simulink subsystem "Subsystem_Driver_DecisionMaker_BAv01"  (R2022b)
settings: Solver=VariableStepAuto  StartTime=0.0  StopTime=10.0  RelTol=1e-3
undefined symbols (not defined in the file): driver, weatherSim
settings Model: Creator=giaco  LastModifiedBy=giaco

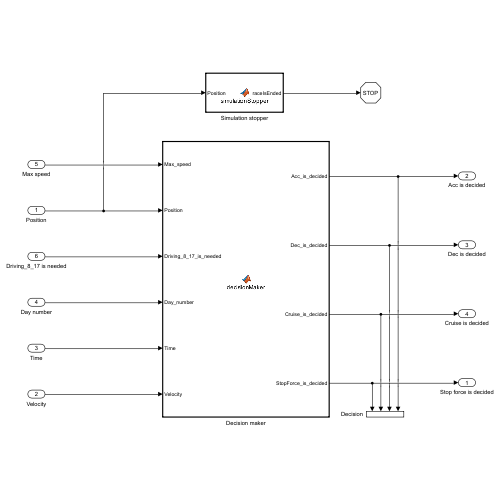
[thumbnail: Simulink's stored preview of the top-level diagram]
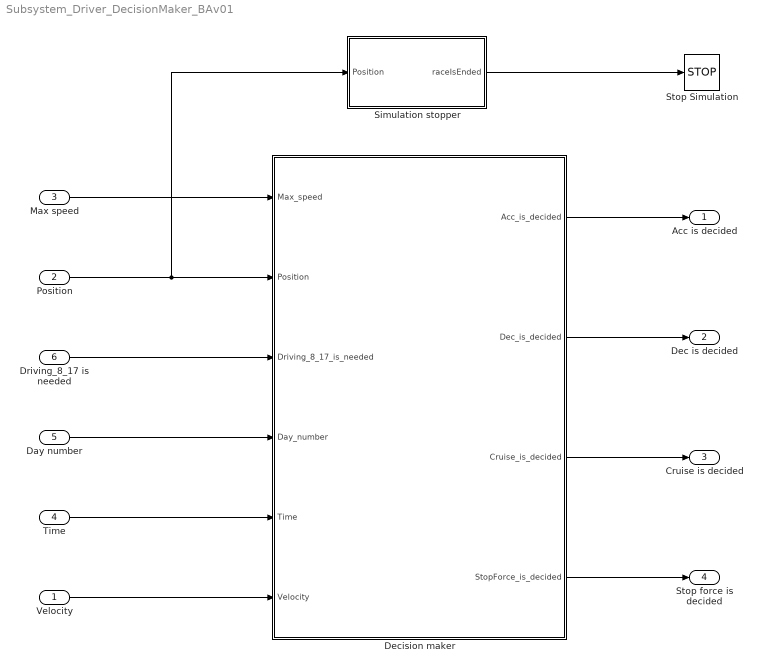
== system Subsystem_Driver_DecisionMaker_BAv01 ==
  Velocity : Inport
  Position : Inport  Port=2
  Max speed : Inport  Port=3
  Time : Inport  Port=4
  Day number : Inport  Port=5
  Driving_8_17 is needed : Inport  Port=6
  Decision maker : MATLAB Function  TreatAsAtomicUnit=on
  Simulation stopper : MATLAB Function  TreatAsAtomicUnit=on
  Stop Simulation : Stop
  Acc is decided : Outport
  Dec is decided : Outport  Port=2
  Cruise is decided : Outport  Port=3
  Stop force is decided : Outport  Port=4  OutDataTypeStr=boolean
  wires:
  Simulation stopper/1(raceIsEnded) -> Stop Simulation/1
  Velocity/1 -> Decision maker/6(Velocity)
  Driving_8_17 is needed/1 -> Decision maker/3(Driving_8_17_is_needed)
  Decision maker/3(Cruise_is_decided) -> Cruise is decided/1
  Position/1 -> Simulation stopper/1(Position), Decision maker/2(Position)
  Decision maker/2(Dec_is_decided) -> Dec is decided/1
  Time/1 -> Decision maker/5(Time)
  Decision maker/4(StopForce_is_decided) -> Stop force is decided/1
  Day number/1 -> Decision maker/4(Day_number)
  Max speed/1 -> Decision maker/1(Max_speed)
  Decision maker/1(Acc_is_decided) -> Acc is decided/1

== matlab function Subsystem_Driver_DecisionMaker_BAv01/Decision maker ==
  settings: updateMethod=DISCRETE
  data: Max_speed input; Position input; Driving_8_17_is_needed input; Day_number input; Time input; Velocity input; spaceStopIsOver data_store_memory; timeStopIsNeeded data_store_memory; spaceStopIsNeeded data_store_memory; driver parameter; spaceStopNumber data_store_memory; spaceStopIsStarted data_store_memory; Acc_is_decided output; Dec_is_decided output; Cruise_is_decided output; StopForce_is_decided output; spaceStopInitialTime data_store_memory; accInitialTime data_store_memory; accInitialVelocity data_store_memory; decInitialTime data_store_memory; decInitialVelocity data_store_memory; racingDayIsStarted data_store_memory; dayNumber data_store_memory; weatherSim parameter
function [Acc_is_decided, Dec_is_decided, Cruise_is_decided, StopForce_is_decided] = decisionMaker(Max_speed, Position, Driving_8_17_is_needed, Day_number, Time, Velocity, driver, weatherSim)

global racingDayIsStarted
global timeStopIsNeeded
global dayNumber

global spaceStopIsNeeded
global spaceStopIsStarted
global spaceStopIsOver
global spaceStopInitialTime
global spaceStopNumber

global accInitialTime
global accInitialVelocity
global decInitialTime
global decInitialVelocity

Acc_is_decided = false;
Dec_is_decided = false;
Cruise_is_decided = false;
StopForce_is_decided = false;

controlVelocity = min(driver.velRef, Max_speed);

%% Check for stops
% Time stops
stopTime = Time - Velocity ./ driver.decRef;

if ~timeStopIsNeeded && stopTime >= (weatherSim.irradiance.stopTimeSec(Day_number) - 60) %to be sure to stop on time
    timeStopIsNeeded = true;
    decInitialTime = Time; %initialization of time and velocity for ramp controller
    decInitialVelocity = Velocity;
end % if

% Space stops
stopDistance = Position - Velocity.^2 / (2 * driver.decRef);

if ~spaceStopIsNeeded && stopDistance >= driver.stopLocDist(spaceStopNumber)
    spaceStopIsNeeded = true;
    decInitialTime = Time; %initialization of time and velocity for ramp controller
    decInitialVelocity = Velocity;
    
    if spaceStopNumber < length(driver.stopLocDist) %omit last stop: stop simulation
        spaceStopNumber = spaceStopNumber + 1;
    end % if
end % if

%% Check for new racing day
if Driving_8_17_is_needed && Day_number == dayNumber
    racingDayIsStarted = true;
    timeStopIsNeeded = false;
    dayNumber = dayNumber + 1;
end % if

%% Select control options
%% Deceleration
if timeStopIsNeeded
    if Velocity > driver.velRefStop
        Dec_is_decided = true;
    else %if Velocity <= driver.velRefStop
        StopForce_is_decided = true;
        Dec_is_decided = false;
    end % if

elseif spaceStopIsNeeded
    if spaceStopIsStarted
        spaceStopDuration = Time - spaceStopInitialTime;
        if spaceStopDuration >= 30*60
            spaceStopIsNeeded = false;
            spaceStopIsStarted = false;
            spaceStopIsOver = true;
            Acc_is_decided = true;
            accInitialTime = Time;
            accInitialVelocity = Velocity;
        else
            StopForce_is_decided = true;
        end % if
    else
        if Velocity > driver.velRefStop
            Dec_is_decided = true;
        else %if Velocity < driver.velRefStop
            spaceStopIsStarted = true;
            spaceStopInitialTime = Time;
            StopForce_is_decided = true;
        end % if
    end % if

%% Acceleration
elseif racingDayIsStarted
    if Velocity < 0.9 * controlVelocity
        Acc_is_decided = true;
    else %if Velocity >= 0.9 * controlVelocity
        Cruise_is_decided = true;
        racingDayIsStarted = false;
    end % if

elseif spaceStopIsOver
    if Velocity < 0.9 * controlVelocity
        Acc_is_decided = true;
    else %if Velocity >= 0.9 * controlVelocity
        Cruise_is_decided = true;
        spaceStopIsOver = false;
    end % if

else
    Cruise_is_decided = true;
end % if

== matlab function Subsystem_Driver_DecisionMaker_BAv01/Simulation stopper ==
  data: Position input; raceIsEnded output; driver parameter
function raceIsEnded = simulationStopper(Position, driver)

raceIsEnded = false;

if Position >= driver.finishLocDist
    raceIsEnded = true;
end % if
